simulink model "s12_euler_fvm_radiation_boundary_ref"  (R2026a)
settings: Solver=VariableStepAuto
model workspace (MAT data in the model file):
  S12_Rad_A = [0  1; -1  -2]
  S12_Rad_B = [0; 1]
  S12_Rad_C = [-1 -0.5]
  S12_Rad_D = 0
  S12_Rad_OutgoingPressure = 14
  S12_Rad_State = [1e-08; -1e-05]
settings Model: Creator=Jovi  LastModifiedBy=Jovi

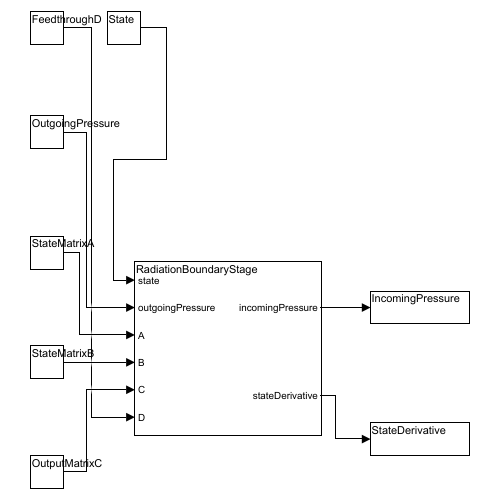
[thumbnail: Simulink's stored preview of the top-level diagram]
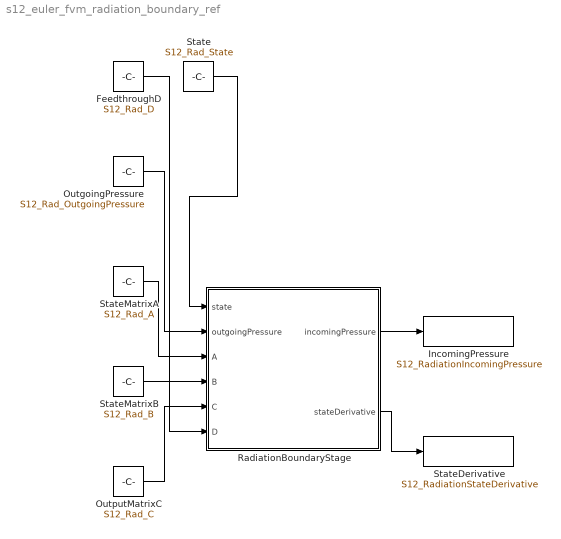
== system s12_euler_fvm_radiation_boundary_ref ==
  FeedthroughD : Constant  Value=S12_Rad_D
  IncomingPressure : ToWorkspace  VariableName=S12_RadiationIncomingPressure
  OutgoingPressure : Constant  Value=S12_Rad_OutgoingPressure
  OutputMatrixC : Constant  Value=S12_Rad_C
  RadiationBoundaryStage : MATLAB Function  TreatAsAtomicUnit=on
  State : Constant  Value=S12_Rad_State
  StateDerivative : ToWorkspace  VariableName=S12_RadiationStateDerivative
  StateMatrixA : Constant  Value=S12_Rad_A
  StateMatrixB : Constant  Value=S12_Rad_B
  wires:
  State/1 -> RadiationBoundaryStage/1(state)
  OutgoingPressure/1 -> RadiationBoundaryStage/2(outgoingPressure)
  StateMatrixA/1 -> RadiationBoundaryStage/3(A)
  StateMatrixB/1 -> RadiationBoundaryStage/4(B)
  OutputMatrixC/1 -> RadiationBoundaryStage/5(C)
  FeedthroughD/1 -> RadiationBoundaryStage/6(D)
  RadiationBoundaryStage/1(incomingPressure) -> IncomingPressure/1
  RadiationBoundaryStage/2(stateDerivative) -> StateDerivative/1

== matlab function s12_euler_fvm_radiation_boundary_ref/RadiationBoundaryStage ==
  data: state input; incomingPressure output; outgoingPressure input; A input; B input; C input; D input; stateDerivative output
function [incomingPressure,stateDerivative] = RadiationBoundaryStage(state,outgoingPressure,A,B,C,D)
%#codegen
stateDerivative = [A(1)*state(1) + A(3)*state(2) + B(1)*outgoingPressure; A(2)*state(1) + A(4)*state(2) + B(2)*outgoingPressure];
incomingPressure = C(1)*state(1) + C(2)*state(2) + D*outgoingPressure;
end
